simulink model "Test1"  (R2019b)
settings: Solver=VariableStepAuto  StartTime=0.0  StopTime=10.0  RelTol=1e-3
settings Model: Creator=Administrator  LastModifiedBy=Administrator

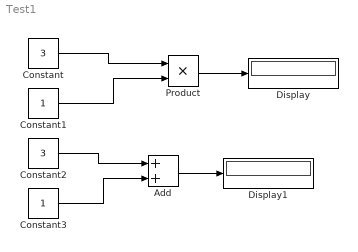
== system Test1 ==
  Add : Sum
  Constant : Constant  Value=3
  Constant1 : Constant
  Constant2 : Constant  Value=3
  Constant3 : Constant
  Display : Display
  Display1 : Display
  Product : Product
  wires:
  Constant/1 -> Product/1
  Constant1/1 -> Product/2
  Product/1 -> Display/1
  Constant2/1 -> Add/1
  Constant3/1 -> Add/2
  Add/1 -> Display1/1
